simulink model "controller"  (R2018a)
settings: Solver=FixedStepDiscrete  StartTime=0.0  StopTime=1  RelTol=1e-3
libraries: powerlib x8
settings Model: Creator=enes_  LastModifiedBy=enes_

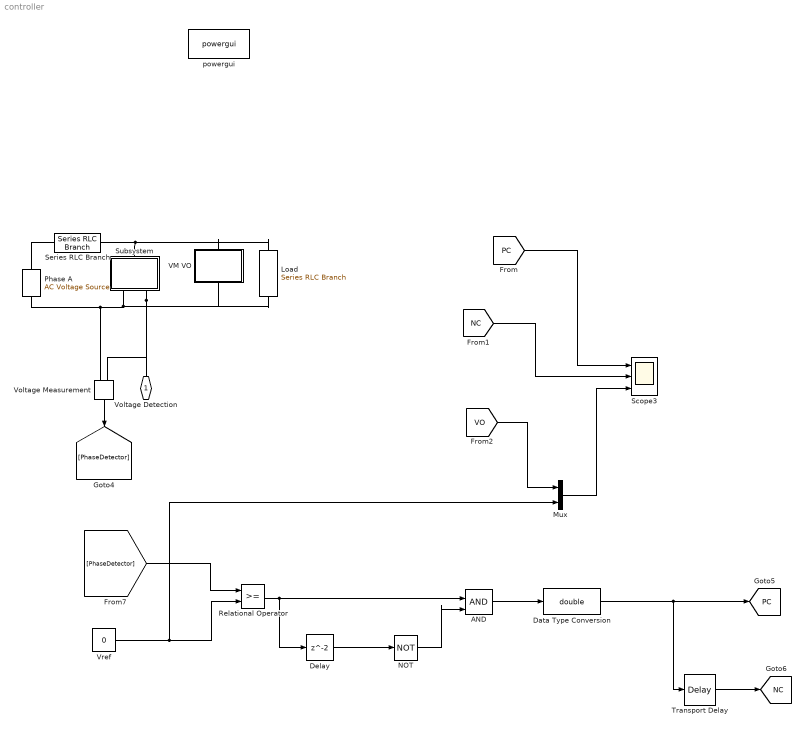
== system controller ==
  AND : Logic  IconShape=distinctive  AllPortsSameDT=off  OutDataTypeStr=boolean
  Data Type Conversion : DataTypeConversion  OutDataTypeStr=double
  Delay : Delay
  Load : powerlib/Elements/Series RLC Branch  LConnTagsString=__new0  RConnTagsString=__new0  BranchType=R  Resistance=15  Inductance=10e-9  SetiL0=off  InitialCurrent=0  Capacitance=1e-6  Setx0=off  InitialVoltage=0  Measurements=None
  Mux : Mux  Inputs=2
  NOT : Logic  Operator=NOT  IconShape=distinctive  AllPortsSameDT=off  OutDataTypeStr=boolean
  Phase A : powerlib/Electrical Sources/AC Voltage Source  Amplitude=230*sqrt(2)  Phase=0  Frequency=50  SampleTime=0  Measurements=None  BusType=swing  Pref=10e3  Qref=0  Qmin=-inf  Qmax=+inf
  Relational Operator : RelationalOperator  OutDataTypeStr=boolean  RndMeth=Simplest
  Scope3 : Scope  NumInputPorts=3
  Series RLC Branch : powerlib/Elements/Series RLC Branch  LConnTagsString=__new0  RConnTagsString=__new0  BranchType=L  Resistance=1  Inductance=5e-3  SetiL0=off  InitialCurrent=0  Capacitance=1e-6  Setx0=off  InitialVoltage=0  Measurements=None
  Subsystem : Subsystem
  Transport Delay : TransportDelay  DelayTime=0.01
  VM VO : Subsystem
  Voltage Measurement : powerlib/Measurements/Voltage Measurement  PhasorSimulation=off  OutputType=Complex  PSBequivalent=0
  Vref : Constant  Value=0
  powergui : powerlib/powergui  Priority=1  SimulationMode=Discrete  SampleTime=1e-6  frequency=60  Iterations=50  frequencyindice=50  Pbase=100e6  ErrMax=1e-4  UnitsV=kV  UnitsW=MW  buscounter=0  FunctionMessages=off  echomessages=off  EnableUseOfTLC=off  CurrentSourceSwitches=off  DisableSnubberDevices=off  DisableRonSwitches=off  DisableVfSwitches=off  DisplayEquations=off  SolverType=Tustin/Backward Euler (TBE)  Interpol=off  ExternalGateDelay=off  methode=off  Ts=100  x0status=blocks  SPID=off  SwTol=0  HookPort=off  RestoreLinks=warning  ResistiveCurrentMeasurement=off  Frange=[0:2:500]  Ylog=off  Xlog=on  ShowGrid=off  save=off  variable=ZData  structure=InputCurrent  ZoomFFT=off  StartTime=2.5  cycles=100  DisplayStyle=2  fundamental=50  FreqAxis=off  MaxFrequency=1000  frequencyindicesteady=1  RmsSteady=1  display=off
  Voltage Detection : PMIOPort  Side=Left
  tag scope: NC=global, PC=global
  wires:
  Voltage Measurement/1 -> [PhaseDetector]
  Delay/1 -> NOT/1
  NOT/1 -> AND/2
  [PhaseDetector] -> Relational Operator/1
  Relational Operator/1 -> Delay/1, AND/1
  Transport Delay/1 -> [NC]
  Vref/1 -> Relational Operator/2, Mux/2
  AND/1 -> Data Type Conversion/1
  [PC] -> Scope3/1
  [NC] -> Scope3/2
  Data Type Conversion/1 -> Transport Delay/1, [PC]
  [VO] -> Mux/1
  Mux/1 -> Scope3/3
  connections:
  Subsystem/LConn1 -- VM VO/LConn1 -- Load/LConn1 -- Series RLC Branch/RConn1
  Subsystem/RConn2 -- Voltage Detection/RConn1 -- Voltage Measurement/LConn1
  Subsystem/RConn1 -- VM VO/RConn1 -- Load/RConn1 -- Phase A/LConn1 -- Voltage Measurement/LConn2
  Phase A/RConn1 -- Series RLC Branch/LConn1

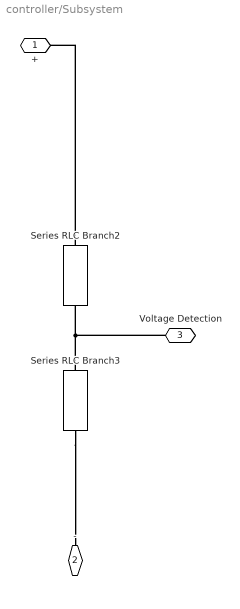
== system controller/Subsystem ==
  Series RLC Branch2 : powerlib/Elements/Series RLC Branch  LConnTagsString=__new0  RConnTagsString=__new0  BranchType=R  Resistance=64e3  Inductance=10e-9  SetiL0=off  InitialCurrent=0  Capacitance=1e-6  Setx0=off  InitialVoltage=0  Measurements=None
  Series RLC Branch3 : powerlib/Elements/Series RLC Branch  LConnTagsString=__new0  RConnTagsString=__new0  BranchType=R  Resistance=1e3  Inductance=10e-9  SetiL0=off  InitialCurrent=0  Capacitance=1e-6  Setx0=off  InitialVoltage=0  Measurements=None
  + : PMIOPort  Side=Left
  - : PMIOPort  Port=2  Side=Right
  Voltage Detection : PMIOPort  Port=3  Side=Right
  connections:
  Series RLC Branch3/LConn1 -- Series RLC Branch2/RConn1 -- Voltage Detection/RConn1
  Series RLC Branch2/LConn1 -- +/RConn1
  Series RLC Branch3/RConn1 -- -/RConn1

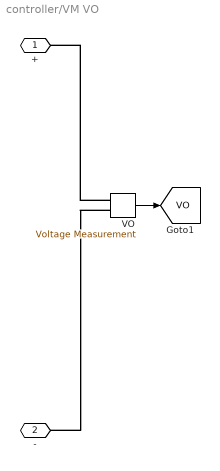
== system controller/VM VO ==
  VO : powerlib/Measurements/Voltage Measurement  PhasorSimulation=off  OutputType=Complex  PSBequivalent=0
  + : PMIOPort  Side=Left
  - : PMIOPort  Port=2  Side=Right
  tag scope: VO=global
  wires:
  VO/1 -> [VO]
  connections:
  VO/LConn2 -- -/RConn1
  VO/LConn1 -- +/RConn1
